simulink model "ECE3331LAB2SLX2CONFIG3"  (R2018a)
settings: Solver=VariableStepAuto  StartTime=0.0  StopTime=10.0  RelTol=1e-3
settings Model: Creator=zshang3  LastModifiedBy=zshang3

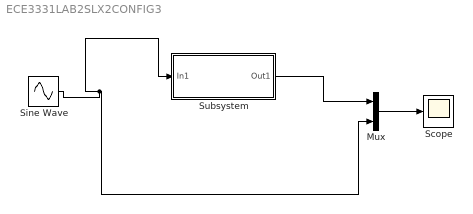
== system ECE3331LAB2SLX2CONFIG3 ==
  Mux : Mux  Inputs=2
  Scope : Scope
  Sine Wave : Sin  SampleTime=0
  Subsystem : Subsystem
  wires:
  Sine Wave/1 -> Mux/2, Subsystem/1(In1)
  Mux/1 -> Scope/1
  Subsystem/1(Out1) -> Mux/1

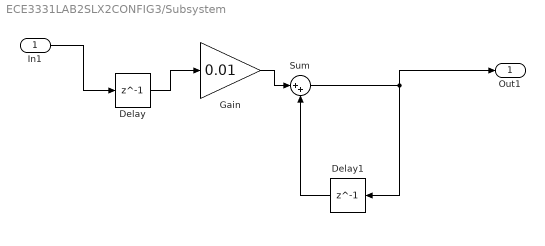
== system ECE3331LAB2SLX2CONFIG3/Subsystem ==
  In1 : Inport
  Delay : Delay  DelayLength=1  InitialCondition=0
  Delay1 : Delay  DelayLength=1  InitialCondition=0
  Gain : Gain  Gain=0.01
  Sum : Sum  Inputs=|++
  Out1 : Outport
  wires:
  Gain/1 -> Sum/1
  Sum/1 -> Out1/1, Delay1/1
  In1/1 -> Delay/1
  Delay/1 -> Gain/1
  Delay1/1 -> Sum/2
